simulink model "SCADA"  (R2025a)
settings: Solver=FixedStepAuto  StartTime=0.0  StopTime=inf  FixedStep=0.001  RelTol=1e-3
InitFcn:
  | addpath('SCADA');
  | initFcn_SCADA;
model workspace (MAT data in the model file):
  RadSysCoeff : Simulink.Parameter (value not decoded)
undefined symbols (not defined in the file): daq, g, HIL_act_A_cap, HIL_act_A_rod, HIL_charge_ki, HIL_charge_kp, HIL_charge_nMax, HIL_charge_nMin, HIL_ERU_kd, HIL_ERU_ki, HIL_ERU_kp, HIL_ERU_nMax, HIL_gen_kd, HIL_gen_ki, HIL_gen_kp, HIL_gen_nMax, HIL_gen_nMin, HIL_H1T_kd, HIL_H1T_ki, HIL_H1T_kp, HIL_H1T_P1fBias, HIL_H1T_P1negCutIn, HIL_H1T_P1posCutIn, HIL_H1T_P2fBias, HIL_H1T_P2negCutIn, HIL_H1T_P2posCutIn, HIL_scale_sys, HIL_WECpump_A_cap, HIL_WECpump_A_rod, HIL_WECpump_ang2lin, HIL_WECpump_negativeCtrlLimit, HIL_WECpump_positiveCtrlLimit, National_Instruments, PCIe, rho, wave_phi, wave_S_w, WEC_A_rad, WEC_B_rad, WEC_dw, WEC_F_amp, WEC_h, WEC_I, WEC_I_inf, WEC_ICs, WEC_L_cm, WEC_L_flap, WEC_m, WEC_phi_e, WEC_T, WEC_W, WEC_w
libraries: sldrtlib x26, slpidlib x4, daqlib x1, simulink x1
(part 2 of 2)

== system SCADA/Sensing/Flow meters ==
  Analog Input1 : sldrtlib/Analog Input  SampleTime=0.1  MaxMissedTicks=10  ShowMissedTicks=off  YieldWhenWaiting=on  DrvName=National_Instruments/PCIe-6343  DrvAddress=4294967295  DrvOptions=[0 528767 48128 3 3 3 3]  Channels=7  RangeMode=1  VoltRange=1  DataType=1
      settings: AttributesFormatString=National Instruments\nPCIe-6343 [auto]
  Analog Input6 : sldrtlib/Analog Input  SampleTime=0.1  MaxMissedTicks=10  ShowMissedTicks=off  YieldWhenWaiting=on  DrvName=National_Instruments/PCIe-6343  DrvAddress=4294967295  DrvOptions=[0 528767 48128 3 3 3 3]  Channels=7  RangeMode=1  VoltRange=1  DataType=1
      settings: AttributesFormatString=National Instruments\nPCIe-6343 [auto]
  Constant1 : Constant  Value=-8.8225e6
  Constant7 : Constant  Value=-8.8225e6
  Gain1 : Gain  Gain=-4.6366e06
  Gain6 : Gain  Gain=-4.6366e6
  Sum1 : Sum  Inputs=|++
  Sum6 : Sum  Inputs=|++
  FM-01 (m3/s) : Outport
  FM-02 (m3/s) : Outport  Port=2
  wires:
  Constant7/1 -> Sum6/2
  Gain6/1 -> Sum6/1
  Sum6/1 -> FM-01 (m3/s)/1
  Gain1/1 -> Sum1/1
  Sum1/1 -> FM-02 (m3/s)/1
  Constant1/1 -> Sum1/2
  Analog Input6/1 -> Gain6/1
  Analog Input1/1 -> Gain1/1

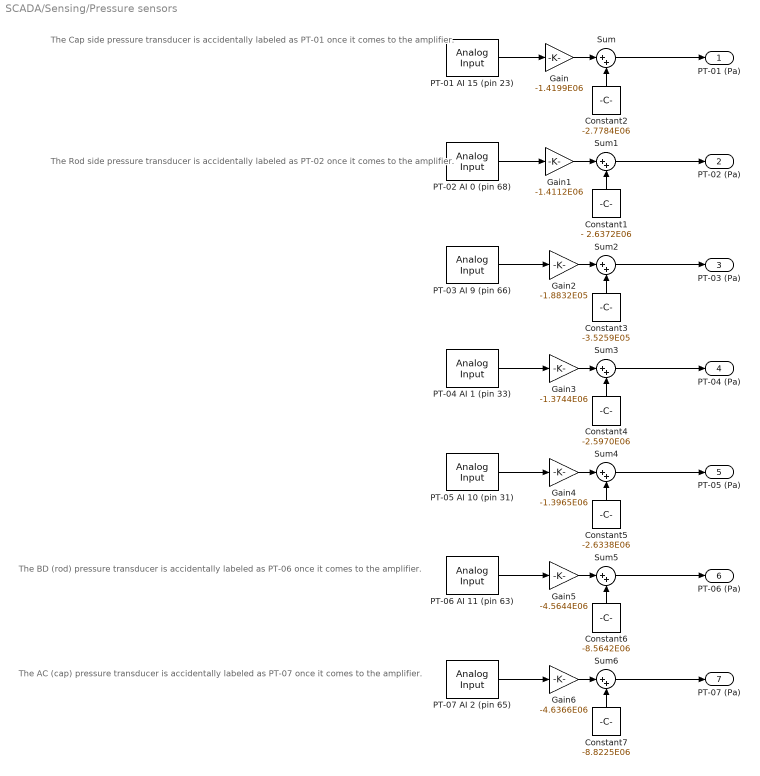
== system SCADA/Sensing/Pressure sensors ==
  note: The Cap side pressure transducer is accidentally labeled as PT-01 once it comes to the amplifier.
  note: The Rod side pressure transducer is accidentally labeled as PT-02 once it comes to the amplifier.
  note: The BD (rod) pressure transducer is accidentally labeled as PT-06 once it comes to the amplifier.
  note: The AC (cap) pressure transducer is accidentally labeled as PT-07 once it comes to the amplifier.
  Constant1 : Constant  Value=- 2.6372E06
  Constant2 : Constant  Value=-2.7784E06
  Constant3 : Constant  Value=-3.5259E05
  Constant4 : Constant  Value=-2.5970E06
  Constant5 : Constant  Value=-2.6338E06
  Constant6 : Constant  Value=-8.5642E06
  Constant7 : Constant  Value=-8.8225E06
  Gain : Gain  Gain=-1.4199E06
  Gain1 : Gain  Gain=-1.4112E06
  Gain2 : Gain  Gain=-1.8832E05
  Gain3 : Gain  Gain=-1.3744E06
  Gain4 : Gain  Gain=-1.3965E06
  Gain5 : Gain  Gain=-4.5644E06
  Gain6 : Gain  Gain=-4.6366E06
  PT-01 AI 15 (pin 23) : sldrtlib/Analog Input  SampleTime=0.001  MaxMissedTicks=inf  ShowMissedTicks=off  YieldWhenWaiting=on  DrvName=National_Instruments/PCIe-6343  DrvAddress=4294967295  DrvOptions=[0 528767 48128 3 3 3 3]  Channels=16  RangeMode=1  VoltRange=1  DataType=1
      settings: AttributesFormatString=National Instruments\nPCIe-6343 [auto]
  PT-02 AI 0 (pin 68) : sldrtlib/Analog Input  SampleTime=0.1  MaxMissedTicks=inf  ShowMissedTicks=off  YieldWhenWaiting=on  DrvName=National_Instruments/PCIe-6343  DrvAddress=4294967295  DrvOptions=[0 528767 48128 3 3 3 3]  Channels=1  RangeMode=1  VoltRange=1  DataType=1
      settings: AttributesFormatString=National Instruments\nPCIe-6343 [auto]
  PT-03 AI 9 (pin 66) : sldrtlib/Analog Input  SampleTime=0.1  MaxMissedTicks=inf  ShowMissedTicks=off  YieldWhenWaiting=on  DrvName=National_Instruments/PCIe-6343  DrvAddress=4294967295  DrvOptions=[0 528767 48128 3 3 3 3]  Channels=10  RangeMode=1  VoltRange=1  DataType=1
      settings: AttributesFormatString=National Instruments\nPCIe-6343 [auto]
  PT-04 AI 1 (pin 33) : sldrtlib/Analog Input  SampleTime=0.1  MaxMissedTicks=10  ShowMissedTicks=off  YieldWhenWaiting=on  DrvName=National_Instruments/PCIe-6343  DrvAddress=4294967295  DrvOptions=[0 528767 48128 3 3 3 3]  Channels=2  RangeMode=1  VoltRange=1  DataType=1
      settings: AttributesFormatString=National Instruments\nPCIe-6343 [auto]
  PT-05 AI 10 (pin 31) : sldrtlib/Analog Input  SampleTime=0.1  MaxMissedTicks=inf  ShowMissedTicks=off  YieldWhenWaiting=on  DrvName=National_Instruments/PCIe-6343  DrvAddress=4294967295  DrvOptions=[0 528767 48128 3 3 3 3]  Channels=11  RangeMode=1  VoltRange=1  DataType=1
      settings: AttributesFormatString=National Instruments\nPCIe-6343 [auto]
  PT-06 AI 11 (pin 63) : sldrtlib/Analog Input  SampleTime=0.1  MaxMissedTicks=10  ShowMissedTicks=off  YieldWhenWaiting=on  DrvName=National_Instruments/PCIe-6343  DrvAddress=4294967295  DrvOptions=[0 528767 48128 3 3 3 3]  Channels=12  RangeMode=1  VoltRange=1  DataType=1
      settings: AttributesFormatString=National Instruments\nPCIe-6343 [auto]
  PT-07 AI 2 (pin 65) : sldrtlib/Analog Input  SampleTime=0.1  MaxMissedTicks=10  ShowMissedTicks=off  YieldWhenWaiting=on  DrvName=National_Instruments/PCIe-6343  DrvAddress=4294967295  DrvOptions=[0 528767 48128 3 3 3 3]  Channels=3  RangeMode=1  VoltRange=1  DataType=1
      settings: AttributesFormatString=National Instruments\nPCIe-6343 [auto]
  Sum{,1..6} (7 alike) : Sum  Inputs=|++
  PT-01 (Pa) : Outport
  PT-02 (Pa) : Outport  Port=2
  PT-03 (Pa) : Outport  Port=3
  PT-04 (Pa) : Outport  Port=4
  PT-05 (Pa) : Outport  Port=5
  PT-06 (Pa) : Outport  Port=6
  PT-07 (Pa) : Outport  Port=7
  wires:
  PT-01 AI 15 (pin 23)/1 -> Gain/1
  Constant2/1 -> Sum/2
  Sum/1 -> PT-01 (Pa)/1
  Sum1/1 -> PT-02 (Pa)/1
  Sum2/1 -> PT-03 (Pa)/1
  Sum3/1 -> PT-04 (Pa)/1
  Sum4/1 -> PT-05 (Pa)/1
  Sum5/1 -> PT-06 (Pa)/1
  Gain/1 -> Sum/1
  PT-02 AI 0 (pin 68)/1 -> Gain1/1
  Constant1/1 -> Sum1/2
  Gain1/1 -> Sum1/1
  PT-03 AI 9 (pin 66)/1 -> Gain2/1
  Constant3/1 -> Sum2/2
  Gain2/1 -> Sum2/1
  PT-04 AI 1 (pin 33)/1 -> Gain3/1
  Constant4/1 -> Sum3/2
  Gain3/1 -> Sum3/1
  PT-05 AI 10 (pin 31)/1 -> Gain4/1
  Constant5/1 -> Sum4/2
  Gain4/1 -> Sum4/1
  PT-06 AI 11 (pin 63)/1 -> Gain5/1
  Constant6/1 -> Sum5/2
  Gain5/1 -> Sum5/1
  PT-07 AI 2 (pin 65)/1 -> Gain6/1
  Sum6/1 -> PT-07 (Pa)/1
  Constant7/1 -> Sum6/2
  Gain6/1 -> Sum6/1

== system SCADA/Sensing/WEC-driven pump position ==
  Analog Input : sldrtlib/Analog Input  SampleTime=0.1  MaxMissedTicks=inf  ShowMissedTicks=off  YieldWhenWaiting=on  DrvName=National_Instruments/PCIe-6343  DrvAddress=4294967295  DrvOptions=[0 528767 48128 3 3 3 3]  Channels=8  RangeMode=1  VoltRange=1  DataType=1
      settings: AttributesFormatString=National Instruments\nPCIe-6343 [auto]
  Constant2 : Constant  Value=0.254
  Gain : Gain  Gain=0.0991
  Scope : Scope
      settings: ActiveDisplayYMinimum=0.18549072799337207  ActiveDisplayYMaximum=0.20028666260571121  DataLoggingVariableName=ScopeData18
  Scope1 : Scope
      settings: ActiveDisplayYMinimum=-0.30249608869568  ActiveDisplayYMaximum=-0.27211161021147162  DataLoggingVariableName=ScopeData19
  Scope2 : Scope
      settings: ActiveDisplayYMinimum=-0.00957891157171476  ActiveDisplayYMaximum=0.10067713496811365  DataLoggingVariableName=ScopeData20
  Sum : Sum  Inputs=|+-
  Pos. meas. (m) : Outport
  wires:
  Constant2/1 -> Sum/2
  Gain/1 -> Scope1/1, Sum/1
  Analog Input/1 -> Scope/1, Gain/1
  Sum/1 -> Scope2/1, Pos. meas. (m)/1

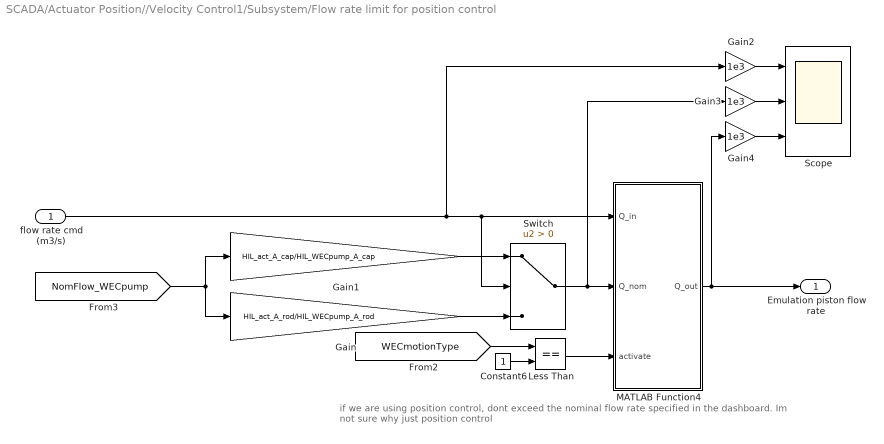
== system SCADA/Actuator Position//Velocity Control1/Subsystem/Flow rate limit for position control ==
  note: if we are using position control, dont exceed the nominal flow rate specified in the dashboard. Im not sure why just position control
  flow rate cmd (m3/s) : Inport
  Constant6 : Constant
  Gain : Gain  Gain=HIL_act_A_rod/HIL_WECpump_A_rod
  Gain1 : Gain  Gain=HIL_act_A_cap/HIL_WECpump_A_cap
  Gain2 : Gain  Gain=1e3
  Gain3 : Gain  Gain=1e3
  Gain4 : Gain  Gain=1e3
  Less Than : RelationalOperator  Operator===  OutDataTypeStr=boolean  RndMeth=Simplest  InputSameDT=off
  MATLAB Function4 : MATLAB Function  TreatAsAtomicUnit=on
  Scope : Scope  NumInputPorts=3
      settings: ActiveDisplayYMinimum=0.67014336374685324  ActiveDisplayYMaximum=1.3156485017885247  DataLoggingSaveFormat=Array
  Switch : Switch  Criteria=u2 > Threshold  SaturateOnIntegerOverflow=off  InputSameDT=off
  Emulation piston flow rate : Outport
  wires:
  Constant6/1 -> Less Than/2
  MATLAB Function4/1(Q_out) -> Gain4/1, Emulation piston flow rate/1
  Switch/1 -> Gain3/1, MATLAB Function4/2(Q_nom)
  Less Than/1 -> MATLAB Function4/3(activate)
  [WECmotionType] -> Less Than/1
  Gain/1 -> Switch/3
  Gain1/1 -> Switch/1
  [NomFlow_WECpump] -> Gain1/1, Gain/1
  flow rate cmd (m3/s)/1 -> Gain2/1, Switch/2, MATLAB Function4/1(Q_in)
  Gain2/1 -> Scope/1
  Gain3/1 -> Scope/2
  Gain4/1 -> Scope/3

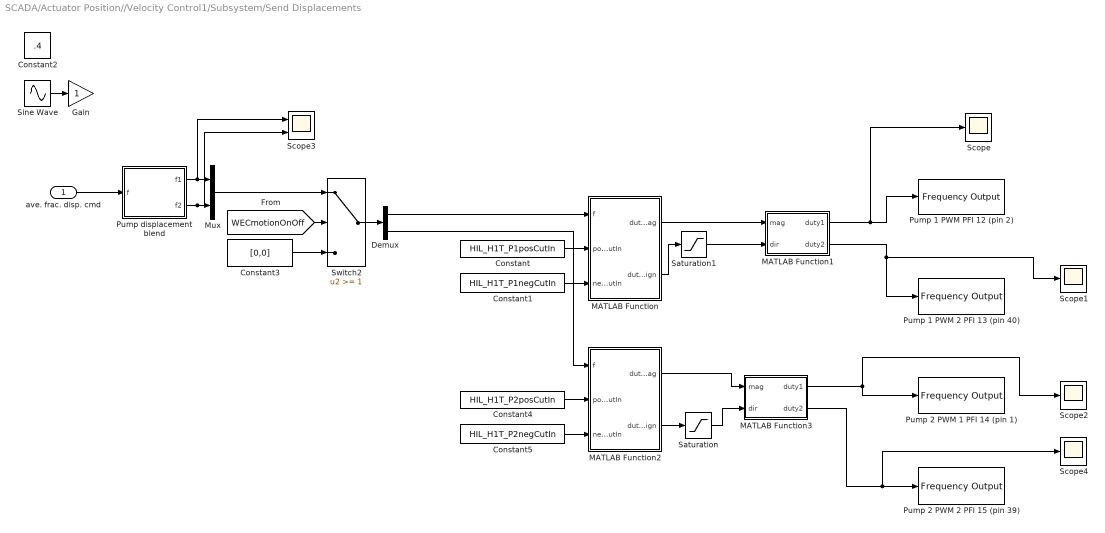
== system SCADA/Actuator Position//Velocity Control1/Subsystem/Send Displacements ==
  ave. frac. disp. cmd : Inport
  Constant : Constant  Value=HIL_H1T_P1posCutIn
  Constant1 : Constant  Value=HIL_H1T_P1negCutIn
  Constant2 : Constant  Value=.4
  Constant3 : Constant  Value=[0,0]
  Constant4 : Constant  Value=HIL_H1T_P2posCutIn
  Constant5 : Constant  Value=HIL_H1T_P2negCutIn
  Demux : Demux  Outputs=2
  Gain : Gain
  MATLAB Function : MATLAB Function  TreatAsAtomicUnit=on
  MATLAB Function1 : MATLAB Function  TreatAsAtomicUnit=on
  MATLAB Function2 : MATLAB Function  TreatAsAtomicUnit=on
  MATLAB Function3 : MATLAB Function  TreatAsAtomicUnit=on
  Mux : Mux  Inputs=2
  Pump 1 PWM PFI 12 (pin 2) : sldrtlib/Frequency Output  SampleTime=0.1  MaxMissedTicks=inf  ShowMissedTicks=off  YieldWhenWaiting=off  DrvName=National_Instruments/PCIe-6343  DrvAddress=4294967295  DrvOptions=[0 528767 48128 3 3 3 3]  Channels=1  FrequencySource=1  Frequency=100  FrequencyFinalValue=[]  DutySource=2  Duty=0  DutyFinalValue=0
      settings: AttributesFormatString=National Instruments\nPCIe-6343 [auto]
  Pump 1 PWM 2 PFI 13 (pin 40) : sldrtlib/Frequency Output  SampleTime=0.1  MaxMissedTicks=inf  ShowMissedTicks=off  YieldWhenWaiting=off  DrvName=National_Instruments/PCIe-6343  DrvAddress=4294967295  DrvOptions=[0 528767 48128 3 3 3 3]  Channels=2  FrequencySource=1  Frequency=100  FrequencyFinalValue=[]  DutySource=2  Duty=0  DutyFinalValue=0
      settings: AttributesFormatString=National Instruments\nPCIe-6343 [auto]
  Pump 2 PWM 1 PFI 14 (pin 1) : sldrtlib/Frequency Output  SampleTime=0.1  MaxMissedTicks=inf  ShowMissedTicks=off  YieldWhenWaiting=off  DrvName=National_Instruments/PCIe-6343  DrvAddress=4294967295  DrvOptions=[0 528767 48128 3 3 3 3]  Channels=3  FrequencySource=1  Frequency=100  FrequencyFinalValue=[]  DutySource=2  Duty=0  DutyFinalValue=0
      settings: AttributesFormatString=National Instruments\nPCIe-6343 [auto]
  Pump 2 PWM 2 PFI 15 (pin 39) : sldrtlib/Frequency Output  SampleTime=0.1  MaxMissedTicks=inf  ShowMissedTicks=off  YieldWhenWaiting=off  DrvName=National_Instruments/PCIe-6343  DrvAddress=4294967295  DrvOptions=[0 528767 48128 3 3 3 3]  Channels=4  FrequencySource=1  Frequency=100  FrequencyFinalValue=[]  DutySource=2  Duty=0  DutyFinalValue=0
      settings: AttributesFormatString=National Instruments\nPCIe-6343 [auto]
  Pump displacement blend : MATLAB Function  TreatAsAtomicUnit=on
  Saturation : Saturate  UpperLimit=1  LowerLimit=0
  Saturation1 : Saturate  UpperLimit=1  LowerLimit=0
  Scope{,1..2,4} (4 alike) : Scope
      Scope settings: ActiveDisplayYMinimum=-1  ActiveDisplayYMaximum=1  DataLoggingVariableName=ScopeData29
      Scope1 settings: ActiveDisplayYMinimum=-1  ActiveDisplayYMaximum=1  DataLoggingVariableName=ScopeData30
      Scope2 settings: ActiveDisplayYMinimum=-1  ActiveDisplayYMaximum=1  DataLoggingVariableName=ScopeData31
      Scope4 settings: ActiveDisplayYMinimum=-1  ActiveDisplayYMaximum=1  DataLoggingVariableName=ScopeData32
  Scope3 : Scope  NumInputPorts=2
      settings: ActiveDisplayYMinimum=-2.25  ActiveDisplayYMaximum=10.25  DataLoggingVariableName=ScopeData24
  Sine Wave : Sin  Amplitude=.1  Frequency=2*pi/10  SampleTime=0
  Switch2 : Switch  Threshold=1  SaturateOnIntegerOverflow=off  InputSameDT=off
  wires:
  MATLAB Function2/1(dutyMag) -> MATLAB Function3/1(mag)
  MATLAB Function/2(dutySign) -> Saturation1/1
  Constant/1 -> MATLAB Function/2(posCutIn)
  Mux/1 -> Switch2/1
  Saturation1/1 -> MATLAB Function1/2(dir)
  Pump displacement blend/2(f2) -> Scope3/2, Mux/2
  Switch2/1 -> Demux/1
  Constant3/1 -> Switch2/3
  Demux/2 -> MATLAB Function2/1(f)
  MATLAB Function2/2(dutySign) -> Saturation/1
  Constant4/1 -> MATLAB Function2/2(posCutIn)
  Demux/1 -> MATLAB Function/1(f)
  Constant1/1 -> MATLAB Function/3(negCutIn)
  Pump displacement blend/1(f1) -> Scope3/1, Mux/1
  Constant5/1 -> MATLAB Function2/3(negCutIn)
  [WECmotionOnOff] -> Switch2/2
  Sine Wave/1 -> Gain/1
  MATLAB Function1/1(duty1) -> Scope/1, Pump 1 PWM PFI 12 (pin 2)/1
  MATLAB Function1/2(duty2) -> Pump 1 PWM 2 PFI 13 (pin 40)/1, Scope1/1
  MATLAB Function/1(dutyMag) -> MATLAB Function1/1(mag)
  Saturation/1 -> MATLAB Function3/2(dir)
  MATLAB Function3/1(duty1) -> Pump 2 PWM 1 PFI 14 (pin 1)/1, Scope2/1
  MATLAB Function3/2(duty2) -> Scope4/1, Pump 2 PWM 2 PFI 15 (pin 39)/1
  ave. frac. disp. cmd/1 -> Pump displacement blend/1(f)

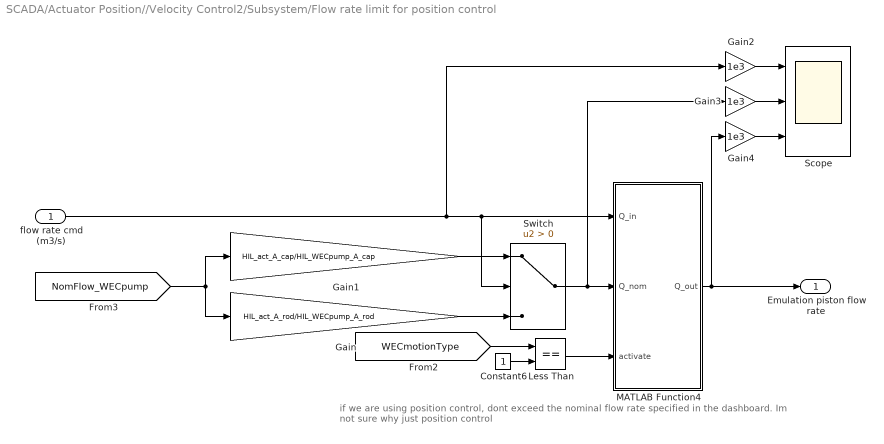
== system SCADA/Actuator Position//Velocity Control2/Subsystem/Flow rate limit for position control ==
  note: if we are using position control, dont exceed the nominal flow rate specified in the dashboard. Im not sure why just position control
  flow rate cmd (m3/s) : Inport
  Constant6 : Constant
  Gain : Gain  Gain=HIL_act_A_rod/HIL_WECpump_A_rod
  Gain1 : Gain  Gain=HIL_act_A_cap/HIL_WECpump_A_cap
  Gain2 : Gain  Gain=1e3
  Gain3 : Gain  Gain=1e3
  Gain4 : Gain  Gain=1e3
  Less Than : RelationalOperator  Operator===  OutDataTypeStr=boolean  RndMeth=Simplest  InputSameDT=off
  MATLAB Function4 : MATLAB Function  TreatAsAtomicUnit=on
  Scope : Scope  NumInputPorts=3
      settings: ActiveDisplayYMinimum=0.67014336374685324  ActiveDisplayYMaximum=1.3156485017885247  DataLoggingSaveFormat=Array
  Switch : Switch  Criteria=u2 > Threshold  SaturateOnIntegerOverflow=off  InputSameDT=off
  Emulation piston flow rate : Outport
  wires:
  Gain4/1 -> Scope/3
  Gain3/1 -> Scope/2
  Gain2/1 -> Scope/1
  flow rate cmd (m3/s)/1 -> MATLAB Function4/1(Q_in), Switch/2, Gain2/1
  [NomFlow_WECpump] -> Gain/1, Gain1/1
  Gain1/1 -> Switch/1
  Gain/1 -> Switch/3
  [WECmotionType] -> Less Than/1
  Less Than/1 -> MATLAB Function4/3(activate)
  Switch/1 -> MATLAB Function4/2(Q_nom), Gain3/1
  MATLAB Function4/1(Q_out) -> Emulation piston flow rate/1, Gain4/1
  Constant6/1 -> Less Than/2

== matlab function SCADA/Actuator Position//Velocity Control1/Subsystem/Send Displacements/MATLAB Function1 ==
  data: mag input; duty1 output; dir input; duty2 output
function [duty1,duty2] = fcn(mag,dir)

if dir == 1
    duty1 = mag;
    duty2 = 0;
else
    duty1 = 0;
    duty2 = mag;   
end

== matlab function SCADA/Actuator Position//Velocity Control1/Subsystem/Send Displacements/MATLAB Function3 ==
  data: mag input; duty1 output; dir input; duty2 output
function [duty1,duty2] = fcn(mag,dir)

if dir == 1
    duty1 = mag;
    duty2 = 0;
else
    duty1 = 0;
    duty2 = mag;   
end

== matlab function SCADA/Motor//Generator Control/RO feed pressure control/Feed forward ==
  data: p input; shaftSpeed_ff output; HIL_charge_cn parameter
function shaftSpeed_ff = fcn(p,HIL_charge_cn)

shaftSpeed_ff = 60*swrt((p-1.013e5)/HIL_charge_cn);

== matlab function SCADA/Actuator Position//Velocity Control1/Subsystem/Flow rate limit for position control/MATLAB Function4 ==
  data: Q_in input; Q_out output; Q_nom input; activate input
function Q_out = fcn(Q_in,Q_nom,activate)
Q_out = Q_in ...
    + (sign(Q_in)*Q_nom - Q_in) * (abs(Q_in) >= Q_nom) * activate;

== matlab function SCADA/Actuator Position//Velocity Control1/Subsystem/Send Displacements/MATLAB Function ==
  data: f input; dutyMag output; dutySign output; posCutIn input; negCutIn input
function [dutyMag,dutySign] = fcn(f,posCutIn, negCutIn)
duty = ((1-posCutIn)*f + posCutIn)*(f>0) + ...
    ((1-negCutIn)*f - negCutIn)*(f<0);
duty = max(-1,min(1,duty));
dutyMag = abs(duty);
dutySign = sign(duty);

== matlab function SCADA/Actuator Position//Velocity Control1/Subsystem/MATLAB Function1 ==
  data: speed_rpm input; maxFlow_m3perSec output; numPumps input; HIL_H1T_D parameter
function maxFlow_m3perSec = fcn(speed_rpm,numPumps,HIL_H1T_D)
eff_vol = 0.92;
displacement = HIL_H1T_D*(0.01)^3; % [cc/rev -> m^3/rev]
maxFlow_m3perSec = numPumps*eff_vol*speed_rpm/60*displacement;

== matlab function SCADA/Actuator Position//Velocity Control1/Subsystem/Send Displacements/MATLAB Function2 ==
  data: f input; dutyMag output; dutySign output; posCutIn input; negCutIn input
function [dutyMag,dutySign] = fcn(f,posCutIn, negCutIn)
duty = ((1-posCutIn)*f + posCutIn)*(f>0) + ...
    ((1-negCutIn)*f - negCutIn)*(f<0);
duty = max(-1,min(1,duty));
dutyMag = abs(duty);
dutySign = sign(duty);

== matlab function SCADA/Actuator Position//Velocity Control1/Subsystem/Send Displacements/Pump displacement blend ==
  data: f input; f1 output; f2 output; HIL_H1T_P1fBias parameter; HIL_H1T_P2fBias parameter
function [f1,f2] = fcn(f,HIL_H1T_P1fBias, HIL_H1T_P2fBias)
    P1 = -HIL_H1T_P1fBias;
    P2 = HIL_H1T_P2fBias;
    
    f1 = (1/(1+P1))*(f-P1) * (f<=P1) ...
       + (2*P2/(P2-P1))*(f-P1) * ((P1 < f) & (f < P2)) ...
       + ((1-2*P2)/(1-P2)*f + 1 - (1-2*P2)/(1-P2)) * (f>=P2);
    
    f2 = ((1+2*P1)/(1+P1)*f + (1+2*P1)/(1+P1) - 1) * (f<=P1) ...
       + (2*P1/(P1-P2))*(f-P2) * ((P1 < f) & (f < P2)) ...
       + (1/(1-P2))*(f-P2) * (f>=P2);

== stateflow chart SCADA/Prescribed Motion/Constant WEC-driven Pump Flow1/State Transition Table ==
  state forward
    entry:
    direction=1;
  state reverse
    entry:
    direction=0;
  (default) -> forward
  forward -> (junction 25) [order 2] : [pos<HIL_WECpump_positiveCtrlLimit]
  (junction 25) -> forward
  forward -> reverse [order 1] : [pos>=HIL_WECpump_positiveCtrlLimit]
  reverse -> forward [order 1] : [pos<=HIL_WECpump_negativeCtrlLimit]
  reverse -> (junction 29) [order 2] : [pos>HIL_WECpump_negativeCtrlLimit]
  (junction 29) -> reverse
  data: pos input; direction output; HIL_WECpump_positiveCtrlLimit parameter; HIL_WECpump_negativeCtrlLimit parameter

== matlab function SCADA/Prescribed Motion/Prescribed Wave-like Motion/Wave-like motion ==
  data: t input; pos output; meanFlow input; w input; WECmotionType input; HIL_WECpump_A_cap parameter; HIL_WECpump_A_rod parameter
function pos = fcn(t,meanFlow,...
                w,WECmotionType,HIL_WECpump_A_cap, HIL_WECpump_A_rod)

% switch WECmotionType
%     case {0,1} % regular motion
        x_amp = meanFlow*pi/2/w/(HIL_WECpump_A_cap + HIL_WECpump_A_rod);
        
        pos = x_amp*sin(w*t);

%     case 1 % irregular motion
%         
%         pos = sum( x_amp.*sin(w.*t + psi));

% end

== matlab function SCADA/WEC Simulation1/Hydrostatic force ==
  data: pos input; T_h output; waveElev input; WEC_L_flap parameter; WEC_h parameter; WEC_T parameter; WEC_W parameter; rho parameter; g parameter; WEC_L_cm parameter; WEC_m parameter
function T_h = fcn(pos,waveElev,...
                    WEC_L_flap,WEC_h,WEC_T,WEC_W,rho, g, WEC_L_cm, WEC_m)
%% Determine buoyant torque from submerged volume

% Height of top edge of flap from hinge
h_top = WEC_L_flap*cos(pos);

% Length of submerged part of plate (by centerline) centroids 
% from thin plate assumption
L_sub = (h_top > WEC_h+waveElev)*(WEC_h+waveElev)/cos(pos) + ...
    (h_top <= WEC_h+waveElev)*WEC_L_flap; 

% Calculate the centroid of the buoyant force, position perpendicular to
% gravity
centroid_x = L_sub/2*sin(pos);

% calculate bouyant torque
T_buoy = WEC_T*L_sub*WEC_W*rho*g*centroid_x;

%% Determine torque due to off center weight
% Calculate position of the center of mass of the flap, perpendicular to
% gravity
cm_x = WEC_L_cm*sin(pos);

% calculate torque due to weight
T_weight = WEC_m*g*cm_x;

%% Determine total effective torque
T_h = T_buoy - T_weight;

== matlab function SCADA/WEC Simulation1/Irregular Waves ==
  data: t input; waveElev output; T_e output; WEC_F_amp parameter; WEC_w parameter; WEC_dw parameter; WEC_phi_e parameter; wave_S_w parameter; wave_phi parameter
function [waveElev,T_e] = fcn(t, WEC_F_amp, WEC_w, WEC_dw, WEC_phi_e, wave_S_w, wave_phi)

T_e = sum( WEC_F_amp.*sqrt(2*wave_S_w.*WEC_dw) ...
            .*sin(WEC_w*t + wave_phi + WEC_phi_e ));

waveElev = sum( sqrt(2*wave_S_w(:).*WEC_dw) ...
                .*sin(WEC_w(:)*t + wave_phi(:)) );

== matlab function SCADA/WEC Simulation1/Regular Waves ==
  data: t input; waveElev output; T_e output; WEC_F_amp parameter; WEC_w parameter; WEC_dw parameter; WEC_phi_e parameter; wave_S_w parameter; wave_phi parameter
function [waveElev,T_e] = fcn(t, WEC_F_amp, WEC_w, WEC_dw, WEC_phi_e, wave_S_w, wave_phi)

T_e = sum( WEC_F_amp.*sqrt(2*wave_S_w.*WEC_dw) ...
            .*sin(WEC_w*t + wave_phi + WEC_phi_e ));

waveElev = sum( sqrt(2*wave_S_w(:).*WEC_dw) ...
                .*sin(WEC_w(:)*t + wave_phi(:)) );

== matlab function SCADA/Actuator Position//Velocity Control2/Subsystem/FF flowrate ==
  data: vel input; flowrate output; HIL_act_A_cap parameter; HIL_act_A_rod parameter
function flowrate = fcn(vel,HIL_act_A_cap,HIL_act_A_rod)
flowrate = vel* ...
           (HIL_act_A_cap*(vel>=0) + ...
            HIL_act_A_rod*(vel<0));

== matlab function SCADA/Actuator Position//Velocity Control2/Subsystem/Flow rate limit for position control/MATLAB Function4 ==
  data: Q_in input; Q_out output; Q_nom input; activate input
function Q_out = fcn(Q_in,Q_nom,activate)
Q_out = Q_in ...
    + (sign(Q_in)*Q_nom - Q_in) * (abs(Q_in) >= Q_nom) * activate;

== matlab function SCADA/Actuator Position//Velocity Control2/Subsystem/MATLAB Function ==
  data: f input; dutyMag output; dutySign output; posCutIn input; negCutIn input
function [dutyMag,dutySign] = fcn(f,posCutIn, negCutIn)
duty = ((1-posCutIn)*f + posCutIn)*(f>0) + ...
    ((1-negCutIn)*f - negCutIn)*(f<0);
duty = max(-1,min(1,duty));
dutyMag = abs(duty);
dutySign = sign(duty);

== matlab function SCADA/ERU Control/RO control/feed forward ==
  data: pressure_feed input; shaftSpeedERU output; recoveryRef input
function shaftSpeedERU = fcn(pressure_feed,recoveryRef)
A_perm = 2.57e-12; % [m^3/(N-s)] permeability coeff.
S_perm = 33.6; % [m^3] membrane area
disp_ERUmotor = 9.31*1e-6; % [cc/rev -> m3/rev] motor displacement
effVol = 0.9;

q_perm = S_perm*A_perm*(pressure_feed - 2.7e6 - 101e3);
q_brineTarget = (1 - recoveryRef)*q_perm;

shaftSpeedERU = q_brineTarget/effVol/disp_ERUmotor*60;

== matlab function SCADA/Actuator Position//Velocity Control2/Subsystem/MATLAB Function1 ==
  data: speed_rpm input; maxFlow_m3perSec output; numPumps input; HIL_H1T_D parameter
function maxFlow_m3perSec = fcn(speed_rpm,numPumps,HIL_H1T_D)
eff_vol = 0.92;
displacement = HIL_H1T_D*(0.01)^3; % [cc/rev -> m^3/rev]
maxFlow_m3perSec = numPumps*eff_vol*speed_rpm/60*displacement;

== matlab function SCADA/Actuator Position//Velocity Control2/Subsystem/MATLAB Function2 ==
  data: f input; dutyMag output; dutySign output; posCutIn input; negCutIn input
function [dutyMag,dutySign] = fcn(f,posCutIn, negCutIn)
duty = ((1-posCutIn)*f + posCutIn)*(f>0) + ...
    ((1-negCutIn)*f - negCutIn)*(f<0);
duty = max(-1,min(1,duty));
dutyMag = abs(duty);
dutySign = sign(duty);

== matlab function SCADA/Actuator Position//Velocity Control2/Subsystem/Pump displacement blend ==
  data: f input; f1 output; f2 output; HIL_H1T_P1fBias parameter; HIL_H1T_P2fBias parameter
function [f1,f2] = fcn(f,HIL_H1T_P1fBias, HIL_H1T_P2fBias)
    P1 = -HIL_H1T_P1fBias;
    P2 = HIL_H1T_P2fBias;
    
    f1 = (1/(1+P1))*(f-P1) * (f<=P1) ...
       + (2*P2/(P2-P1))*(f-P1) * ((P1 < f) & (f < P2)) ...
       + ((1-2*P2)/(1-P2)*f + 1 - (1-2*P2)/(1-P2)) * (f>=P2);
    
    f2 = ((1+2*P1)/(1+P1)*f + (1+2*P1)/(1+P1) - 1) * (f<=P1) ...
       + (2*P1/(P1-P2))*(f-P2) * ((P1 < f) & (f < P2)) ...
       + (1/(1-P2))*(f-P2) * (f>=P2);
